simulink model "ThrotModel_FirstPrincChamb_DataDrivenServoValve"  (R2025b)
settings: Solver=FixedStepAuto  StartTime=0.0  StopTime=10.0  FixedStep=.01  RelTol=1e-3
values from neighbouring files (symbols this model uses):
  a = -5    [init_engine_params.m]
  b = 6.7e7    (= 67000000)    [init_engine_params.m]
  C_f = K_f / (rho_f * V_line)    (= 4349372348.87)    [init_engine_params.m]
  C_ox = K_ox / (rho_ox * V_line)    (= 5893224561.79)    [init_engine_params.m]
  CdA_table = [      1.5e-6 ... (first row only)    [init_engine_params.m]
  k_servo = 1    [init_engine_params.m]
  P_1_f = P_tank_f - DeltaP_lines_f    (= 3013637.644)    [init_engine_params.m]
  P_1_ox = P_tank_ox - DeltaP_lines_ox    (= 3012738.487)    [init_engine_params.m]
  P_amb = 101325    [init_engine_params.m]
  P_c_nom = 350 * psi_to_Pa    (= 2413166)    [init_engine_params.m]
  P_c_ref_bp = [             0 ... (first row only)    [init_engine_params.m]
  psi_to_Pa = 6894.76    [init_engine_params.m]
  rho_f = 789    [init_engine_params.m]
  rho_ox = 988.82    [init_engine_params.m]
  tau_servo = 0.05    [init_engine_params.m]
  theta_bp = [       0 ... (first row only)    [init_engine_params.m]
  theta_ff_table = [       0 ... (first row only)    [init_engine_params.m]
undefined symbols (not defined in the file or in its folder): CdA_inj_f, CdA_inj_ox, k_noz
libraries: slpidlib x1
settings Model: Creator=gruby  LastModifiedBy=gruby

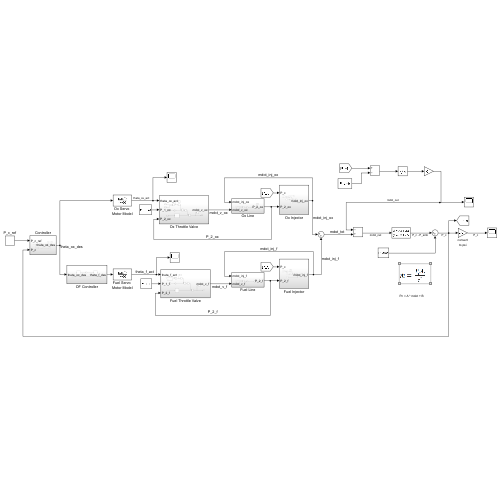
[thumbnail: Simulink's stored preview of the top-level diagram]
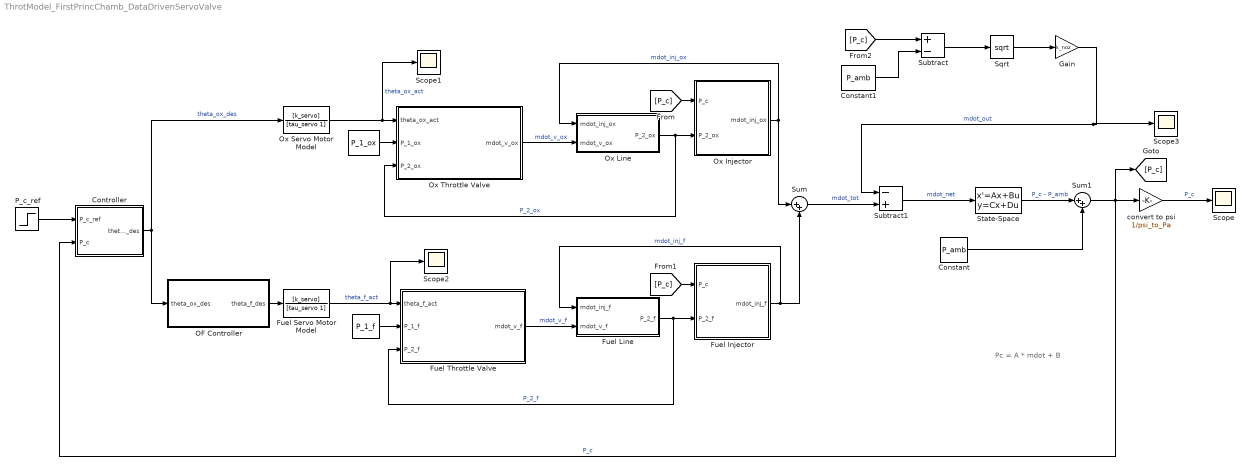
== system ThrotModel_FirstPrincChamb_DataDrivenServoValve ==
  note: Pc = A * mdot + B
  " " : Constant  Value=P_1_ox
  "  " : Constant  Value=P_1_f
  Constant : Constant  Value=P_amb
  Constant1 : Constant  Value=P_amb
  Controller : Subsystem
  Fuel Injector : Subsystem
  Fuel Line : Subsystem
  Fuel Servo Motor Model : TransferFcn  Numerator=[k_servo]  Denominator=[tau_servo 1]
  Fuel Throttle Valve : Subsystem
  Gain : Gain  Gain=k_noz
  OF Controller : Subsystem
  Ox Injector : Subsystem
  Ox Line : Subsystem
  Ox Servo Motor Model : TransferFcn  Numerator=[k_servo]  Denominator=[tau_servo 1]
  Ox Throttle Valve : Subsystem
  P_c_ref : Step  Before=P_amb  After=P_c_nom  SampleTime=0
  Scope{,1..3} (4 alike) : Scope
      Scope settings: ActiveDisplayYMinimum=-652.90625666117433  ActiveDisplayYMaximum=6023.1157400104994
      Scope1 settings: ActiveDisplayYMinimum=-1  ActiveDisplayYMaximum=1  DataLoggingVariableName=ScopeData13
      Scope2 settings: ActiveDisplayYMinimum=-1  ActiveDisplayYMaximum=1  DataLoggingVariableName=ScopeData14
      Scope3 settings: ActiveDisplayYMinimum=-1  ActiveDisplayYMaximum=1  DataLoggingVariableName=ScopeData15
  Sqrt : Sqrt
  State-Space : StateSpace  A=a  B=b  D=0  InitialCondition=0
  Subtract : Sum  Inputs=+-
  Subtract1 : Sum  Inputs=-+
  Sum : Sum  Inputs=|++
  Sum1 : Sum  Inputs=|++
  convert to psi : Gain  Gain=1/psi_to_Pa
  wires:
  Ox Throttle Valve/1(mdot_v_ox) -> Ox Line/2(mdot_v_ox)  "mdot_v_ox"
  Ox Injector/1(mdot_inj_ox) -> Sum/1, Ox Line/1(mdot_inj_ox)  "mdot_inj_ox"
  Fuel Injector/1(mdot_inj_f) -> Sum/2, Fuel Line/1(mdot_inj_f)  "mdot_inj_f"
  Sum/1 -> Subtract1/2  "mdot_tot"
  [P_c] -> Ox Injector/1(P_c)
  [P_c] -> Fuel Injector/1(P_c)
  Ox Line/1(P_2_ox) -> Ox Throttle Valve/3(P_2_ox), Ox Injector/2(P_2_ox)  "P_2_ox"
  Fuel Line/1(P_2_f) -> Fuel Throttle Valve/3(P_2_f), Fuel Injector/2(P_2_f)  "P_2_f"
  " "/1 -> Ox Throttle Valve/2(P_1_ox)
  "  "/1 -> Fuel Throttle Valve/2(P_1_f)
  Fuel Servo Motor Model/1 -> Scope2/1, Fuel Throttle Valve/1(theta_f_act)  "theta_f_act"
  Controller/1(theta_ox_des) -> OF Controller/1(theta_ox_des), Ox Servo Motor Model/1  "theta_ox_des"
  OF Controller/1(theta_f_des) -> Fuel Servo Motor Model/1
  P_c_ref/1 -> Controller/1(P_c_ref)
  Fuel Throttle Valve/1(mdot_v_f) -> Fuel Line/2(mdot_v_f)  "mdot_v_f"
  State-Space/1 -> Sum1/1  "P_c - P_amb"
  Constant/1 -> Sum1/2
  Sum1/1 -> Controller/2(P_c), convert to psi/1, [P_c]  "P_c"
  convert to psi/1 -> Scope/1  "P_c"
  Ox Servo Motor Model/1 -> Scope1/1, Ox Throttle Valve/1(theta_ox_act)  "theta_ox_act"
  Constant1/1 -> Subtract/2
  Subtract/1 -> Sqrt/1
  Sqrt/1 -> Gain/1
  Gain/1 -> Scope3/1, Subtract1/1  "mdot_out"
  Subtract1/1 -> State-Space/1  "mdot_net"
  [P_c] -> Subtract/1

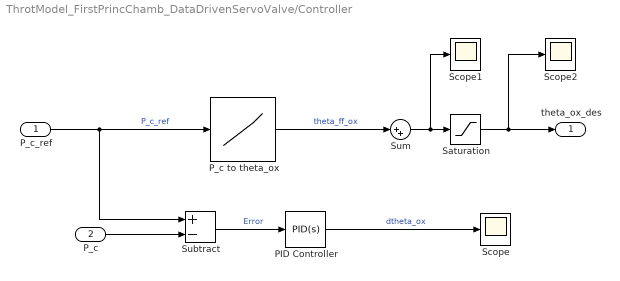
== system ThrotModel_FirstPrincChamb_DataDrivenServoValve/Controller ==
  P_c_ref : Inport
  P_c : Inport  Port=2
  PID Controller : slpidlib/PID Controller  Controller=PID  Form=Parallel  TimeDomain=Continuous-time  UseExternalTs=off  SampleTime=-1  IntegratorMethod=Forward Euler  FilterMethod=Forward Euler  ControllerParametersSource=internal  P=1  I=.1  UseKiTs=off  D=0  UseExternalDerivativeSource=off  N=100  UseFilter=on  TunerSelectOption=Transfer Function Based (PID Tuner App)  InitialConditionSource=internal  InitialConditionForIntegrator=0  InitialConditionForFilter=0  DifferentiatorICPrevScaledInput=0  ExternalReset=none  TrackingMode=off  Kt=1  LimitOutput=off  SatLimitsSource=internal  UpperSaturationLimit=inf  LowerSaturationLimit=-inf  LinearizeAsGain=on  AntiWindupMode=none  Kb=1  LimitIntegrator=off  UpperIntegratorSaturationLimit=inf  LowerIntegratorSaturationLimit=-inf  POutMin=[]  POutMax=[]  IOutMin=[]  IOutMax=[]  DOutMin=[]  DOutMax=[]  NOutMin=[]  NOutMax=[]  SumOutMin=[]  SumOutMax=[]  SaturationOutMin=[]  SaturationOutMax=[]  PParamMin=[]  PParamMax=[]  IParamMin=[]  IParamMax=[]  DParamMin=[]  DParamMax=[]  NParamMin=[]  NParamMax=[]  KbParamMin=[]  KbParamMax=[]  KtParamMin=[]  KtParamMax=[]  KbOutMin=[]  KbOutMax=[]  KtOutMin=[]  KtOutMax=[]  IntegratorOutMin=[]  IntegratorOutMax=[]  FilterOutMin=[]  FilterOutMax=[]  SumI1OutMin=[]  SumI1OutMax=[]  SumI2OutMin=[]  SumI2OutMax=[]  SumI3OutMin=[]  SumI3OutMax=[]  SumI4OutMin=[]  SumI4OutMax=[]  SumDOutMin=[]  SumDOutMax=[]  DifferentiatorOutMin=[]  DifferentiatorOutMax=[]  FilterDiffOutCoefMin=[]  FilterDiffOutCoefMax=[]  ReciprocalOutMin=[]  ReciprocalOutMax=[]  SumDenOutMin=[]  SumDenOutMax=[]  SumNumOutMin=[]  SumNumOutMax=[]  DivideOutMin=[]  DivideOutMax=[]  UdiffTsProdOutMin=[]  UdiffTsProdOutMax=[]  NTsProdOutMin=[]  NTsProdOutMax=[]  UintegralTsProdOutMin=[]  UintegralTsProdOutMax=[]  UngainTsProdOutMin=[]  UngainTsProdOutMax=[]  ClampingZeroOutDataTypeStr=Inherit: Inherit via back propagation  ClampingZeroOutMin=[]  ClampingZeroOutMax=[]  FilterDenConstantOutDataTypeStr=Inherit: Inherit via back propagation  FilterDenConstantOutMin=[]  FilterDenConstantOutMax=[]  PCopyOutDataTypeStr=Inherit: Inherit via back propagation  PCopyOutMin=[]  PCopyOutMax=[]  NCopyOutDataTypeStr=Inherit: Inherit via back propagation  NCopyOutMin=[]  NCopyOutMax=[]  IntegratorContinuousStateAttributes=''  IntegratorStateMustResolveToSignalObject=off  IntegratorRTWStateStorageClass=Auto  FilterContinuousStateAttributes=''  FilterStateMustResolveToSignalObject=off  FilterRTWStateStorageClass=Auto  ParallelPVariant=InternalParameters  IdealPVariant=Disabled  IVariant=InternalParameters  DVariant=InternalParameters  IntegratorVariant=Continuous  SatVariant=Disabled  AWVariant=Passthrough  PCopyVariant=Disabled  TRVariant=Disabled  FdbkBlocksVariant=Forward  IdealPFdbkVariant=Disabled  SatFdbkVariant=Disabled  DerivativeFilterVariant=ContFilter  NVariant=InternalParameters  NCopyVariant=Disabled  FilterICVariant=InternalICsFilter  IntegratorICVariant=InternalICs  ExternalResetVariant=Disabled  TRSumVariant=Passthrough  SumFdbkVariant=Disabled  SumVariant=Sum_PID  TsampFilterVariant=InternalTs  TsampNgainVariant=Passthrough  TsampIntegralVariant=Disabled_SignalSpec  ExternalSaturationOutDataTypeStr=Inherit: Same as second input  DerivativeSourceVariant=ErrorSignal  PreIntVariant=InternalPreInt
  P_c to theta_ox : Lookup_n-D  NumberOfTableDimensions=1  BreakpointsForDimension1=P_c_ref_bp  Table=theta_ff_table  InternalRulePriority=Speed  RndMeth=Simplest
  Saturation : Saturate  UpperLimit=60  LowerLimit=0
  Scope : Scope
      settings: ActiveDisplayYMinimum=-1  ActiveDisplayYMaximum=1  DataLoggingVariableName=ScopeData4
  Scope1 : Scope
      settings: ActiveDisplayYMinimum=1.0265  ActiveDisplayYMaximum=3.0265  DataLoggingVariableName=ScopeData5
  Scope2 : Scope
      settings: ActiveDisplayYMinimum=1.0265  ActiveDisplayYMaximum=3.0265  DataLoggingVariableName=ScopeData7
  Subtract : Sum  Inputs=+-
  Sum : Sum  Inputs=|++
  theta_ox_des : Outport
  wires:
  P_c_ref/1 -> Subtract/1, P_c to theta_ox/1  "P_c_ref"
  P_c to theta_ox/1 -> Sum/1  "theta_ff_ox"
  P_c/1 -> Subtract/2
  Subtract/1 -> PID Controller/1  "Error"
  PID Controller/1 -> Scope/1  "dtheta_ox"
  Sum/1 -> Saturation/1, Scope1/1
  Saturation/1 -> Scope2/1, theta_ox_des/1

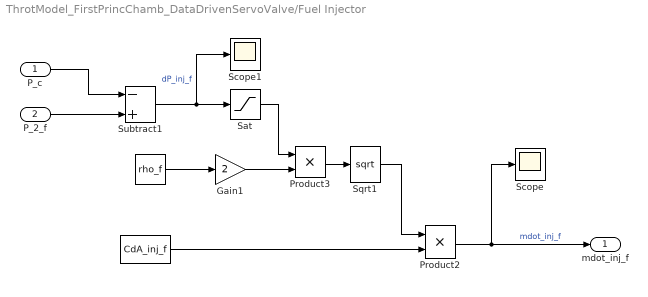
== system ThrotModel_FirstPrincChamb_DataDrivenServoValve/Fuel Injector ==
  P_c : Inport
  P_2_f : Inport  Port=2
  "  " : Constant  Value=CdA_inj_f
  "    " : Constant  Value=rho_f
  Gain1 : Gain  Gain=2
  Product2 : Product
  Product3 : Product
  Sat : Saturate  UpperLimit=+inf  LowerLimit=0
  Scope : Scope
      settings: ActiveDisplayYMinimum=-1  ActiveDisplayYMaximum=1  DataLoggingVariableName=ScopeData8
  Scope1 : Scope
      settings: DataLoggingVariableName=ScopeData9
  Sqrt1 : Sqrt
  Subtract1 : Sum  Inputs=-+
  mdot_inj_f : Outport
  wires:
  Subtract1/1 -> Scope1/1, Sat/1  "dP_inj_f"
  "  "/1 -> Product2/2
  "    "/1 -> Gain1/1
  P_2_f/1 -> Subtract1/2
  Product3/1 -> Sqrt1/1
  Sqrt1/1 -> Product2/1
  Gain1/1 -> Product3/2
  P_c/1 -> Subtract1/1
  Product2/1 -> Scope/1, mdot_inj_f/1  "mdot_inj_f"
  Sat/1 -> Product3/1

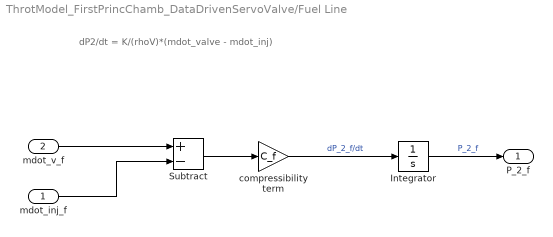
== system ThrotModel_FirstPrincChamb_DataDrivenServoValve/Fuel Line ==
  note: dP2/dt = K/(rhoV)*(mdot_valve - mdot_inj)
  mdot_inj_f : Inport
  mdot_v_f : Inport  Port=2
  Integrator : Integrator  InitialCondition=P_1_f
  Subtract : Sum  Inputs=+-
  compressibility term : Gain  Gain=C_f
  P_2_f : Outport
  wires:
  mdot_v_f/1 -> Subtract/1
  mdot_inj_f/1 -> Subtract/2
  Subtract/1 -> compressibility term/1
  compressibility term/1 -> Integrator/1  "dP_2_f/dt"
  Integrator/1 -> P_2_f/1  "P_2_f"

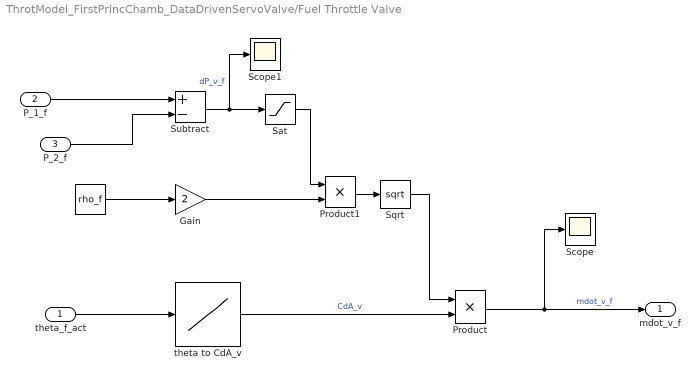
== system ThrotModel_FirstPrincChamb_DataDrivenServoValve/Fuel Throttle Valve ==
  theta_f_act : Inport
  P_1_f : Inport  Port=2
  P_2_f : Inport  Port=3
  "  " : Constant  Value=rho_f
  Gain : Gain  Gain=2
  Product : Product
  Product1 : Product
  Sat : Saturate  UpperLimit=+inf  LowerLimit=0
  Scope : Scope
      settings: DataLoggingVariableName=ScopeData11
  Scope1 : Scope
      settings: ActiveDisplayYMinimum=-1  ActiveDisplayYMaximum=1  DataLoggingVariableName=ScopeData12
  Sqrt : Sqrt
  Subtract : Sum  Inputs=+-
  theta to CdA_v : Lookup_n-D  NumberOfTableDimensions=1  BreakpointsForDimension1=theta_bp  Table=CdA_table  InternalRulePriority=Speed  RndMeth=Simplest
  mdot_v_f : Outport
  wires:
  Subtract/1 -> Scope1/1, Sat/1  "dP_v_f"
  Sqrt/1 -> Product/1
  "  "/1 -> Gain/1
  Product/1 -> Scope/1, mdot_v_f/1  "mdot_v_f"
  Gain/1 -> Product1/2
  theta to CdA_v/1 -> Product/2  "CdA_v"
  Product1/1 -> Sqrt/1
  theta_f_act/1 -> theta to CdA_v/1
  P_2_f/1 -> Subtract/2
  P_1_f/1 -> Subtract/1
  Sat/1 -> Product1/1

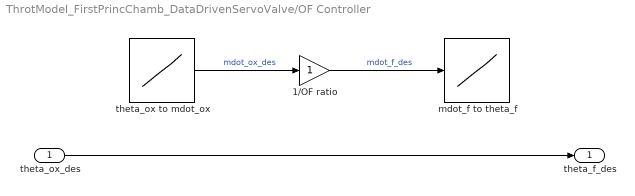
== system ThrotModel_FirstPrincChamb_DataDrivenServoValve/OF Controller ==
  theta_ox_des : Inport
  1/OF ratio : Gain
  mdot_f to theta_f : Lookup_n-D  NumberOfTableDimensions=1  BreakpointsForDimension1=[-5:5]  Table=tanh([-5:5])  InternalRulePriority=Speed  RndMeth=Simplest
  theta_ox to mdot_ox : Lookup_n-D  NumberOfTableDimensions=1  BreakpointsForDimension1=[-5:5]  Table=tanh([-5:5])  InternalRulePriority=Speed  RndMeth=Simplest
  theta_f_des : Outport
  wires:
  theta_ox_des/1 -> theta_f_des/1
  theta_ox to mdot_ox/1 -> 1/OF ratio/1  "mdot_ox_des"
  1/OF ratio/1 -> mdot_f to theta_f/1  "mdot_f_des"

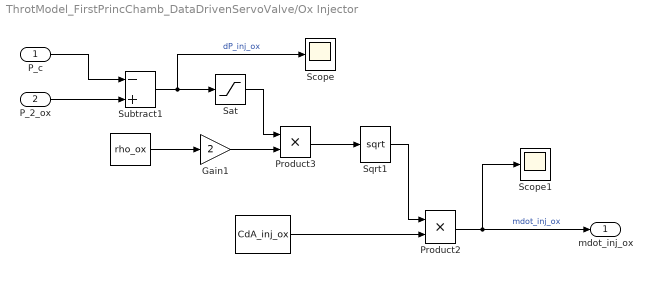
== system ThrotModel_FirstPrincChamb_DataDrivenServoValve/Ox Injector ==
  P_c : Inport
  P_2_ox : Inport  Port=2
  " " : Constant  Value=rho_ox
  "    " : Constant  Value=CdA_inj_ox
  Gain1 : Gain  Gain=2
  Product2 : Product
  Product3 : Product
  Sat : Saturate  UpperLimit=+Inf  LowerLimit=0
  Scope : Scope
      settings: ActiveDisplayYMinimum=-1  ActiveDisplayYMaximum=1
  Scope1 : Scope
      settings: ActiveDisplayYMinimum=-1  ActiveDisplayYMaximum=1  DataLoggingVariableName=ScopeData2
  Sqrt1 : Sqrt
  Subtract1 : Sum  Inputs=-+
  mdot_inj_ox : Outport
  wires:
  Subtract1/1 -> Scope/1, Sat/1  "dP_inj_ox"
  "    "/1 -> Product2/2
  " "/1 -> Gain1/1
  P_2_ox/1 -> Subtract1/2
  Product3/1 -> Sqrt1/1
  Sqrt1/1 -> Product2/1
  Gain1/1 -> Product3/2
  P_c/1 -> Subtract1/1
  Product2/1 -> Scope1/1, mdot_inj_ox/1  "mdot_inj_ox"
  Sat/1 -> Product3/1

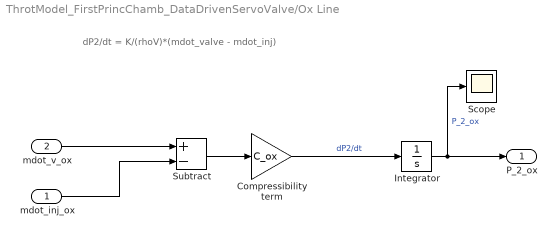
== system ThrotModel_FirstPrincChamb_DataDrivenServoValve/Ox Line ==
  note: dP2/dt = K/(rhoV)*(mdot_valve - mdot_inj)
  mdot_inj_ox : Inport
  mdot_v_ox : Inport  Port=2
  "Compressibility term " : Gain  Gain=C_ox
  Integrator : Integrator  InitialCondition=P_1_ox
  Scope : Scope
      settings: ActiveDisplayYMinimum=-1  ActiveDisplayYMaximum=1  DataLoggingVariableName=ScopeData3
  Subtract : Sum  Inputs=+-
  P_2_ox : Outport
  wires:
  mdot_v_ox/1 -> Subtract/1
  mdot_inj_ox/1 -> Subtract/2
  Subtract/1 -> "Compressibility term "/1
  "Compressibility term "/1 -> Integrator/1  "dP2/dt"
  Integrator/1 -> Scope/1, P_2_ox/1  "P_2_ox"

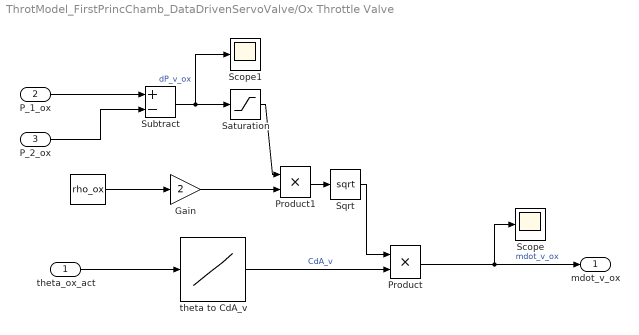
== system ThrotModel_FirstPrincChamb_DataDrivenServoValve/Ox Throttle Valve ==
  theta_ox_act : Inport
  P_1_ox : Inport  Port=2
  P_2_ox : Inport  Port=3
  "  " : Constant  Value=rho_ox
  Gain : Gain  Gain=2
  Product : Product
  Product1 : Product
  Saturation : Saturate  UpperLimit=+inf  LowerLimit=0
  Scope : Scope
      settings: ActiveDisplayYMinimum=-1  ActiveDisplayYMaximum=1  DataLoggingVariableName=ScopeData6
  Scope1 : Scope
      settings: ActiveDisplayYMinimum=-1  ActiveDisplayYMaximum=1  DataLoggingVariableName=ScopeData10
  Sqrt : Sqrt
  Subtract : Sum  Inputs=+-
  theta to CdA_v : Lookup_n-D  NumberOfTableDimensions=1  BreakpointsForDimension1=theta_bp  Table=CdA_table  InternalRulePriority=Speed  RndMeth=Simplest
  mdot_v_ox : Outport
  wires:
  Subtract/1 -> Scope1/1, Saturation/1  "dP_v_ox"
  Sqrt/1 -> Product/1
  "  "/1 -> Gain/1
  Product/1 -> Scope/1, mdot_v_ox/1  "mdot_v_ox"
  Gain/1 -> Product1/2
  theta to CdA_v/1 -> Product/2  "CdA_v"
  Product1/1 -> Sqrt/1
  theta_ox_act/1 -> theta to CdA_v/1
  P_1_ox/1 -> Subtract/1
  P_2_ox/1 -> Subtract/2
  Saturation/1 -> Product1/1
